simulink model "sampleModel2070"  (R2023a)
settings: Solver=VariableStepAuto  StartTime=0.0  StopTime=10.0  RelTol=1e-3
libraries: hdlsllib x4
settings Model: Creator=user1  LastModifiedBy=user1

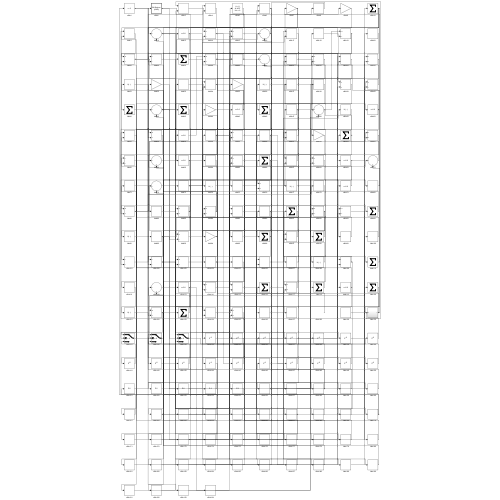
[thumbnail: Simulink's stored preview of the top-level diagram]
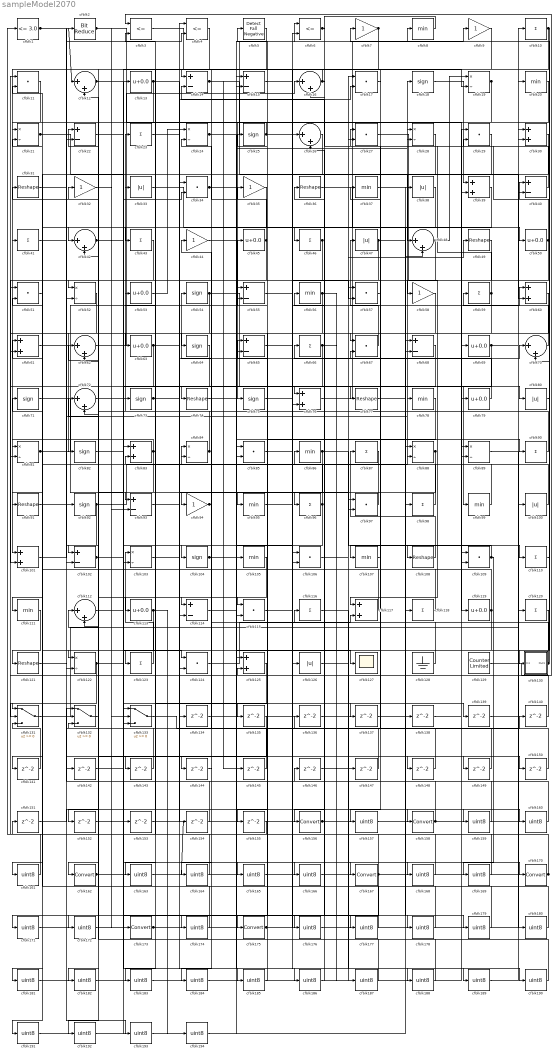
== system sampleModel2070 ==
  cfblk1 : hdlsllib/Logic and Bit Operations/Compare To Constant  relop=<=  const=3.0  OutDataTypeStr=boolean
  cfblk{10,23,41,43,46,59,66,87,90,96,98,110,116,118,120,123} (16 alike) : Sum  Inputs=+
  cfblk{33,38,47,80,100,126} (6 alike) : Abs  SaturateOnIntegerOverflow=off
  cfblk{30,39,60..61,76,83,101,117,125} (9 alike) : Sum
  cfblk{14..15,22,40,55,65,68,93,102,114} (10 alike) : Sum  Inputs=+-
  cfblk{19,21,24,28,52,81,84,88..89,103,122} (11 alike) : Product  Inputs=*/  RndMeth=Zero  SaturateOnIntegerOverflow=on
  cfblk{18,25,54,64,71,73,75,82,92,104} (10 alike) : Signum
  cfblk{8,20,37,56,78,86,95,99,105,107,111} (11 alike) : MinMax
  cfblk{11,17,27,29,34,51,57,67,85,97,106,109,115,124} (14 alike) : DotProduct  OutDataTypeStr=Inherit: Inherit via internal rule
  cfblk{31,36,49,74,77,91,108,121} (8 alike) : Reshape
  cfblk{12,16,26,42,48,62,70,72,112} (9 alike) : Sum  Inputs=|++
  cfblk{13,45,50,53,63,69,79,113,119} (9 alike) : Bias  Bias=0.0  SaturateOnIntegerOverflow=off
  cfblk127 : Scope
  cfblk128 : Ground
  cfblk129 : hdlsllib/Sources/Counter Limited  uplimit=7  tsamp=-1
  cfblk130 : Subsystem
      settings: LibrarySourceBlock=|
      | hdlsllib/Ports &
      | Subsystems/Subsystem
  cfblk131 : Switch  SaturateOnIntegerOverflow=off  InputSameDT=off
  cfblk132 : Switch  SaturateOnIntegerOverflow=off  InputSameDT=off
  cfblk133 : Switch  SaturateOnIntegerOverflow=off  InputSameDT=off
  cfblk{134..155} (22 alike) : Delay  SampleTime=1
  cfblk{156,158,162,167,170,173,175} (7 alike) : DataTypeConversion  SaturateOnIntegerOverflow=off  RndMeth=Floor
  cfblk{157,159..161,163..166,168..169,171..172,174,176..194} (32 alike) : DataTypeConversion  OutDataTypeStr=uint8  SaturateOnIntegerOverflow=off  RndMeth=Floor
  cfblk2 : hdlsllib/Logic and Bit Operations/Bit Reduce  mode=AND
  cfblk3 : RelationalOperator  Operator=<=  OutDataTypeStr=boolean  InputSameDT=off
  cfblk{7,9,32,35,44,58,94} (7 alike) : Gain
  cfblk4 : RelationalOperator  Operator=<=  OutDataTypeStr=boolean  InputSameDT=off
  cfblk5 : hdlsllib/Logic and Bit Operations/Detect Fall Negative  vinit=0  OutDataTypeStr=boolean
  cfblk6 : RelationalOperator  Operator=<=  OutDataTypeStr=boolean  InputSameDT=off
  wires:
  cfblk62/1 -> cfblk16/1
  cfblk104/1 -> cfblk28/2, cfblk174/1
  cfblk18/1 -> cfblk39/1
  cfblk128/1 -> cfblk54/1
  cfblk130/1(Out1) -> cfblk7/1, cfblk66/1
  cfblk84/1 -> cfblk23/1, cfblk31/1
  cfblk76/1 -> cfblk9/1
  cfblk5/1 -> cfblk94/1
  cfblk8/1 -> cfblk75/1
  cfblk123/1 -> cfblk103/1
  cfblk58/1 -> cfblk67/1
  cfblk21/1 -> cfblk103/2, cfblk4/2
  cfblk53/1 -> cfblk24/1
  cfblk16/1 -> cfblk14/1, cfblk96/1
  cfblk7/1 -> cfblk16/2, cfblk22/2
  cfblk97/1 -> cfblk84/1
  cfblk37/1 -> cfblk117/1
  cfblk6/1 -> cfblk76/1, cfblk46/1
  cfblk88/1 -> cfblk113/1, cfblk176/1
  cfblk124/1 -> cfblk117/2
  cfblk12/1 -> cfblk109/1, cfblk19/2, cfblk166/1
  cfblk56/1 -> cfblk115/1, cfblk147/1
  cfblk11/1 -> cfblk101/1
  cfblk67/1 -> cfblk47/1
  cfblk100/1 -> cfblk18/1
  cfblk114/1 -> cfblk8/1
  cfblk19/1 -> cfblk42/1, cfblk114/1
  cfblk34/1 -> cfblk104/1, cfblk150/1
  cfblk3/1 -> cfblk76/2
  cfblk132/1 -> cfblk42/2
  cfblk83/1 -> cfblk81/1, cfblk122/1, cfblk53/1
  cfblk105/1 -> cfblk162/1
  cfblk45/1 -> cfblk35/1, cfblk24/2, cfblk61/2
  cfblk54/1 -> cfblk99/1, cfblk81/2, cfblk106/2
  cfblk24/1 -> cfblk6/1, cfblk90/1
  cfblk98/1 -> cfblk65/1
  cfblk70/1 -> cfblk59/1
  cfblk117/1 -> cfblk5/1
  cfblk108/1 -> cfblk87/1
  cfblk41/1 -> cfblk92/1
  cfblk102/1 -> cfblk124/1, cfblk165/1
  cfblk30/1 -> cfblk48/1
  cfblk75/1 -> cfblk60/1
  cfblk118/1 -> cfblk71/1
  cfblk4/1 -> cfblk41/1
  cfblk1/1 -> cfblk12/1, cfblk193/1
  cfblk120/1 -> cfblk175/1
  cfblk40/1 -> cfblk14/2
  cfblk93/1 -> cfblk70/1
  cfblk119/1 -> cfblk61/1, cfblk141/1
  cfblk36/1 -> cfblk50/1
  cfblk38/1 -> cfblk115/2
  cfblk46/1 -> cfblk111/1, cfblk102/1
  cfblk22/1 -> cfblk74/1
  cfblk96/1 -> cfblk86/1, cfblk133/3
  cfblk9/1 -> cfblk52/1
  cfblk81/1 -> cfblk45/1, cfblk78/1
  cfblk15/1 -> cfblk170/1
  cfblk57/1 -> cfblk37/1
  cfblk61/1 -> cfblk33/1
  cfblk71/1 -> cfblk133/1
  cfblk44/1 -> cfblk127/1
  cfblk82/1 -> cfblk73/1
  cfblk101/1 -> cfblk2/1
  cfblk86/1 -> cfblk110/1, cfblk114/2
  cfblk14/1 -> cfblk60/2, cfblk145/1
  cfblk87/1 -> cfblk83/2
  cfblk66/1 -> cfblk95/1, cfblk172/1, cfblk187/1
  cfblk10/1 -> cfblk63/1, cfblk130/1(In1), cfblk77/1, cfblk102/2
  cfblk63/1 -> cfblk101/2, cfblk185/1
  cfblk94/1 -> cfblk44/1, cfblk144/1
  cfblk32/1 -> cfblk173/1
  cfblk109/1 -> cfblk107/1, cfblk169/1
  cfblk111/1 -> cfblk121/1
  cfblk107/1 -> cfblk27/1
  cfblk35/1 -> cfblk64/1
  cfblk13/1 -> cfblk52/2, cfblk97/2
  cfblk28/1 -> cfblk91/1
  cfblk2/1 -> cfblk119/1, cfblk93/2
  cfblk72/1 -> cfblk167/1
  cfblk48/1 -> cfblk58/1, cfblk19/1
  cfblk50/1 -> cfblk29/2, cfblk93/1
  cfblk113/1 -> cfblk152/1, cfblk194/1
  cfblk129/1 -> cfblk3/1
  cfblk52/1 -> cfblk82/1
  cfblk79/1 -> cfblk36/1
  cfblk42/1 -> cfblk34/2, cfblk133/2, cfblk22/1, cfblk137/1
  cfblk69/1 -> cfblk30/2, cfblk108/1
  cfblk33/1 -> cfblk118/1
  cfblk90/1 -> cfblk62/1
  cfblk20/1 -> cfblk156/1
  cfblk110/1 -> cfblk70/2
  cfblk80/1 -> cfblk40/1
  cfblk59/1 -> cfblk28/1, cfblk143/1
  cfblk95/1 -> cfblk6/2
  cfblk49/1 -> cfblk131/1
  cfblk25/1 -> cfblk21/1, cfblk57/2
  cfblk73/1 -> cfblk80/1, cfblk123/1, cfblk17/2
  cfblk116/1 -> cfblk158/1
  cfblk77/1 -> cfblk98/1
  cfblk106/1 -> cfblk49/1
  cfblk122/1 -> cfblk131/2, cfblk168/1
  cfblk27/1 -> cfblk69/1
  cfblk60/1 -> cfblk124/2
  cfblk65/1 -> cfblk126/1
  cfblk29/1 -> cfblk43/1
  cfblk131/1 -> cfblk10/1
  cfblk47/1 -> cfblk62/2, cfblk179/1
  cfblk92/1 -> cfblk88/2, cfblk122/2, cfblk153/1
  cfblk99/1 -> cfblk21/2
  cfblk103/1 -> cfblk134/1
  cfblk134/1 -> cfblk39/2
  cfblk23/1 -> cfblk135/1
  cfblk136/1 -> cfblk27/2
  cfblk137/1 -> cfblk88/1
  cfblk138/1 -> cfblk109/2
  cfblk115/1 -> cfblk139/1
  cfblk139/1 -> cfblk30/1
  cfblk133/1 -> cfblk140/1
  cfblk140/1 -> cfblk51/1
  cfblk141/1 -> cfblk131/3
  cfblk91/1 -> cfblk142/1
  cfblk143/1 -> cfblk132/3
  cfblk145/1 -> cfblk12/2
  cfblk147/1 -> cfblk132/1
  cfblk121/1 -> cfblk148/1
  cfblk148/1 -> cfblk84/2
  cfblk126/1 -> cfblk149/1
  cfblk149/1 -> cfblk34/1
  cfblk150/1 -> cfblk67/2
  cfblk152/1 -> cfblk48/2
  cfblk153/1 -> cfblk4/1
  cfblk154/1 -> cfblk83/1
  cfblk78/1 -> cfblk155/1
  cfblk155/1 -> cfblk1/1
  cfblk156/1 -> cfblk138/1, cfblk38/1
  cfblk17/1 -> cfblk157/1
  cfblk157/1 -> cfblk20/1
  cfblk158/1 -> cfblk136/1, cfblk132/2
  cfblk31/1 -> cfblk159/1
  cfblk159/1 -> cfblk116/1
  cfblk151/1 -> cfblk160/1
  cfblk160/1 -> cfblk29/1
  cfblk43/1 -> cfblk161/1
  cfblk161/1 -> cfblk151/1
  cfblk162/1 -> cfblk154/1, cfblk40/2
  cfblk64/1 -> cfblk163/1
  cfblk163/1 -> cfblk105/1
  cfblk26/1 -> cfblk164/1
  cfblk164/1 -> cfblk11/1
  cfblk165/1 -> cfblk26/1
  cfblk166/1 -> cfblk26/2
  cfblk167/1 -> cfblk11/2, cfblk171/1
  cfblk168/1 -> cfblk72/1
  cfblk169/1 -> cfblk72/2
  cfblk170/1 -> cfblk3/2, cfblk56/1
  cfblk171/1 -> cfblk15/1
  cfblk172/1 -> cfblk15/2
  cfblk173/1 -> cfblk106/1, cfblk17/1
  cfblk174/1 -> cfblk32/1
  cfblk175/1 -> cfblk65/2, cfblk79/1, cfblk97/1
  cfblk176/1 -> cfblk120/1
  cfblk55/1 -> cfblk177/1
  cfblk177/1 -> cfblk51/2
  cfblk142/1 -> cfblk178/1
  cfblk178/1 -> cfblk55/1
  cfblk179/1 -> cfblk55/2
  cfblk89/1 -> cfblk180/1
  cfblk180/1 -> cfblk25/1
  cfblk39/1 -> cfblk181/1
  cfblk181/1 -> cfblk89/1
  cfblk135/1 -> cfblk182/1
  cfblk182/1 -> cfblk89/2
  cfblk125/1 -> cfblk183/1
  cfblk183/1 -> cfblk57/1
  cfblk144/1 -> cfblk184/1
  cfblk184/1 -> cfblk125/1
  cfblk185/1 -> cfblk125/2
  cfblk112/1 -> cfblk186/1
  cfblk186/1 -> cfblk146/1
  cfblk187/1 -> cfblk112/1
  cfblk74/1 -> cfblk188/1
  cfblk188/1 -> cfblk112/2
  cfblk85/1 -> cfblk189/1
  cfblk189/1 -> cfblk100/1
  cfblk146/1 -> cfblk190/1
  cfblk190/1 -> cfblk85/1
  cfblk51/1 -> cfblk191/1
  cfblk191/1 -> cfblk85/2
  cfblk68/1 -> cfblk192/1
  cfblk192/1 -> cfblk13/1
  cfblk193/1 -> cfblk68/1
  cfblk194/1 -> cfblk68/2

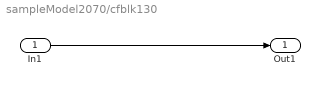
== system sampleModel2070/cfblk130 ==
  In1 : Inport
  Out1 : Outport
  wires:
  In1/1 -> Out1/1
